simulink model "Switch_Block"  (R2023a)
settings: Solver=VariableStepAuto  StartTime=0.0  StopTime=10.0  RelTol=1e-3
settings Model: Creator=Aman  LastModifiedBy=Aman

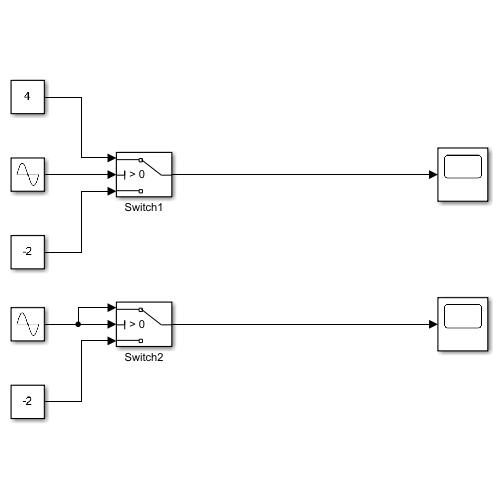
[thumbnail: Simulink's stored preview of the top-level diagram]
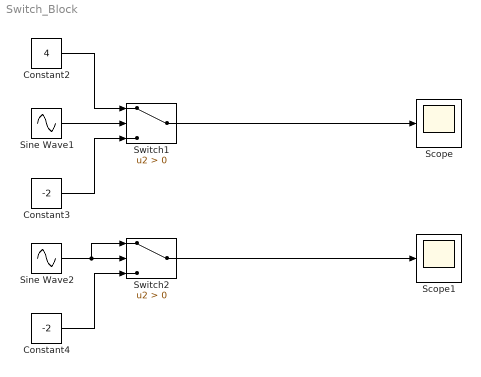
== system Switch_Block ==
  Constant2 : Constant  Value=4
  Constant3 : Constant  Value=-2
  Constant4 : Constant  Value=-2
  Scope : Scope
  Scope1 : Scope
  Sine Wave1 : Sin  SampleTime=0
  Sine Wave2 : Sin  SampleTime=0
  Switch1 : Switch  Criteria=u2 > Threshold  SaturateOnIntegerOverflow=off  InputSameDT=off
  Switch2 : Switch  Criteria=u2 > Threshold  SaturateOnIntegerOverflow=off  InputSameDT=off
  wires:
  Switch1/1 -> Scope/1
  Constant2/1 -> Switch1/1
  Constant3/1 -> Switch1/3
  Sine Wave1/1 -> Switch1/2
  Constant4/1 -> Switch2/3
  Switch2/1 -> Scope1/1
  Sine Wave2/1 -> Switch2/1, Switch2/2
